simulink model "phBopen"  (R2021a)
settings: Solver=VariableStepAuto  StartTime=0.0  StopTime=50  RelTol=1e-3
settings Model: Creator=User  LastModifiedBy=USER
settings SolverCC: AlgebraicLoopSolver=TrustRegion
settings DebuggingCC: SFMachineParentedDataDiag=warning
settings SFSimCC: CustomCodeUndefinedFunction=UseInterfaceOnly

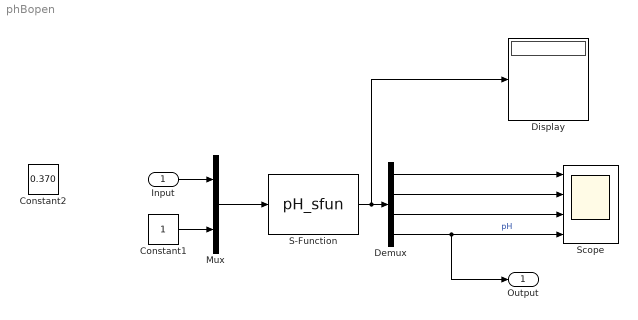
== system phBopen ==
  Input : Inport
  Constant1 : Constant
  Constant2 : Constant  Value=0.370
  Demux : Demux
  Display : Display
  Mux : Mux  Inputs=2
  S-Function : S-Function  FunctionName=pH_sfun  SFunctionDeploymentMode=off  EnableBusSupport=off
  Scope : Scope  NumInputPorts=4
  Output : Outport  VectorParamsAs1DForOutWhenUnconnected=off
  wires:
  Input/1 -> Mux/1
  Constant1/1 -> Mux/2
  Mux/1 -> S-Function/1
  S-Function/1 -> Display/1, Demux/1
  Demux/1 -> Scope/1
  Demux/2 -> Scope/2
  Demux/3 -> Scope/3
  Demux/4 -> Output/1, Scope/4  "pH"
